simulink model "lookup_nD_TestGen33"  (R2017b)
settings: Solver=FixedStepDiscrete  StartTime=0.0  StopTime=10.0  RelTol=1e-3
model workspace (MAT data in the model file):
  LUTObjLKnD33 = Simulink.LookupTable
  LUTObjLKnD33.Table = Simulink.lookuptable.Table
  LUTObjLKnD33.Table.Value = reshape([4 16 10 4 16 10 4 16 10 4 16 10 4 16 10 4 16 10 5 19 18 5 19 18 5 19 18 5 19 18 5 19 18 5 19 18 6 20 23 6 20 23 6 20 23 6 20 23 6 20 23 6 20 23 7 21 24 7 21 24 7 21 24 7 21 24 7 21 24 7 21 24 8 22 25 8 22 25 8 22 25 8 22 25 8 22 25 8 22 25 4 16 10 4 16 10 4 16 10 4 16 10 4 16 10 4 16 10 5 19 18 5 19 18 5 19 18 5 19 18 5 19 18 5 19 18 6 20 23 6 20 23 6 20 23 6 20 23 6 20 23 6 20 23 7 21 24 7 21 24 7 21 24 7 21 24 7 21 24 7 21 24 8 22 25 8 22 25 8 22 25 8 22 25 8 22 25 8 22 25 4 16 10 4 16 10 4 16 10 4 16 10 4 16 10 4 16 10 5 19 18 5 19 18 5 19 18 5 19 18 5 19 18 5 19 18 6 20 23 6 20 23 6 20 23 6 20 23 6 20 23 6 20 23 7 21 24 7 21 24 7 21 24 7 21 24 7 21 24 7 21 24 8 22 25 8 22 25 8 22 25 8 22 25 8 22 25 8 22 25 4 16 10 4 16 10 4 16 10 4 16 10 4 16 10 4 16 10 5 19 18 5 19 18 5 19 18 5 19 18 5 19 18 5 19 18 6 20 23 6 20 23 6 20 23 6 20 23 6 20 23 6 20 23 7 21 24 7 21 24 7 21 24 7 21 24 7 21 24 7 21 24 8 22 25 8 22 25 8 22 25 8 22 25 8 22 25 8 22 25 4 16 10 4 16 10 4 16 10 4 16 10 4 16 10 4 16 10 5 19 18 5 19 18 5 19 18 5 19 18 5 19 18 5 19 18 6 20 23 6 20 23 6 20 23 6 20 23 6 20 23 6 20 23 7 21 24 7 21 24 7 21 24 7 21 24 7 21 24 7 21 24 8 22 25 8 22 25 8 22 25 8 22 25 8 22 25 8 22 25 4 16 10 4 16 10 4 16 10 4 16 10 4 16 10 4 16 10 5 19 18 5 19 18 5 19 18 5 19 18 5 19 18 5 19 18 6 20 23 6 20 23 6 20 23 6 20 23 6 20 23 6 20 23 7 21 24 7 21 24 7 21 24 7 21 24 7 21 24 7 21 24 8 22 25 8 22 25 8 22 25 8 22 25 8 22 25 8 22 25 4 16 10 4 16 10 4 16 10 4 16 10 4 16 10 4 16 10 5 19 18 5 19 18 5 19 18 5 19 18 5 19 18 5 19 18 6 20 23 6 20 23 6 20 23 6 20 23 6 20 23 6 20 23 7 21 24 7 21 24 7 21 24 7 21 24 7 21 24 7 21 24 8 22 25 8 22 25 8 22 25 8 22 25 8 22 25 8 22 25 4 16 10 4 16 10 4 16 10 4 16 10 4 16 10 4 16 10 5 19 18 5 19 18 5 19 18 5 19 18 5 19 18 5 19 18 6 20 23 6 20 23 6 20 23 6 20 23 6 20 23 6 20 23 7 21 24 7 21 24 7 21 24 7 21 24 7 21 24 7 21 24 8 22 25 8 22 25 8 22 25 8 22 25 8 22 25 8 22 25], [2 5 3 2 3 4])
  LUTObjLKnD33.Table.Dimensions = [2 5 3 2 3 4]
  LUTObjLKnD33.Table.DataType = 'double'
  LUTObjLKnD33.Table.FieldName = 'Table'
  LUTObjLKnD33.Breakpoints(1) = Simulink.lookuptable.Breakpoint
  LUTObjLKnD33.Breakpoints(1).Value = [55.1141389852; 115.959753023]
  LUTObjLKnD33.Breakpoints(1).TunableSizeName = 'N1'
  LUTObjLKnD33.Breakpoints(1).Dimensions = [2 1]
  LUTObjLKnD33.Breakpoints(1).DataType = 'double'
  LUTObjLKnD33.Breakpoints(1).FieldName = 'BP1'
  LUTObjLKnD33.Breakpoints(2) = Simulink.lookuptable.Breakpoint
  LUTObjLKnD33.Breakpoints(2).Value = [7.76812849772; 29.4671423139; 31.4118384647; 67.8975675265; 99.4838661864]
  LUTObjLKnD33.Breakpoints(2).TunableSizeName = 'N2'
  LUTObjLKnD33.Breakpoints(2).Dimensions = [5 1]
  LUTObjLKnD33.Breakpoints(2).DataType = 'double'
  LUTObjLKnD33.Breakpoints(2).FieldName = 'BP2'
  LUTObjLKnD33.Breakpoints(3) = Simulink.lookuptable.Breakpoint
  LUTObjLKnD33.Breakpoints(3).Value = [61.8687772676; 86.0025709843; 101.597469424]
  LUTObjLKnD33.Breakpoints(3).TunableSizeName = 'N3'
  LUTObjLKnD33.Breakpoints(3).Dimensions = [3 1]
  LUTObjLKnD33.Breakpoints(3).DataType = 'double'
  LUTObjLKnD33.Breakpoints(3).FieldName = 'BP3'
  LUTObjLKnD33.Breakpoints(4) = Simulink.lookuptable.Breakpoint
  LUTObjLKnD33.Breakpoints(4).Value = [45.1909970892; 88.5981999607]
  LUTObjLKnD33.Breakpoints(4).TunableSizeName = 'N4'
  LUTObjLKnD33.Breakpoints(4).Dimensions = [2 1]
  LUTObjLKnD33.Breakpoints(4).DataType = 'double'
  LUTObjLKnD33.Breakpoints(4).FieldName = 'BP4'
  LUTObjLKnD33.Breakpoints(5) = Simulink.lookuptable.Breakpoint
  LUTObjLKnD33.Breakpoints(5).Value = [48.7941996351; 67.4387180631; 70.5577350792]
  LUTObjLKnD33.Breakpoints(5).TunableSizeName = 'N5'
  LUTObjLKnD33.Breakpoints(5).Dimensions = [3 1]
  LUTObjLKnD33.Breakpoints(5).DataType = 'double'
  LUTObjLKnD33.Breakpoints(5).FieldName = 'BP5'
  LUTObjLKnD33.Breakpoints(6) = Simulink.lookuptable.Breakpoint
  LUTObjLKnD33.Breakpoints(6).Value = [9.10881332364; 75.0691190596; 86.3387833349; 95.4088639299]
  LUTObjLKnD33.Breakpoints(6).TunableSizeName = 'N6'
  LUTObjLKnD33.Breakpoints(6).Dimensions = [4 1]
  LUTObjLKnD33.Breakpoints(6).DataType = 'double'
  LUTObjLKnD33.Breakpoints(6).FieldName = 'BP6'
  LUTObjLKnD33.SupportTunableSize = 0
  LUTObjLKnD33.StructTypeInfo = Simulink.lookuptable.StructTypeInfo
  LUTObjLKnD33.StructTypeInfo.Name = 'LUT'
  LUTObjLKnD33.StructTypeInfo.DataScope = 'Auto'
settings Model: Creator=ktrinh  LastModifiedBy=ktrinh
settings DebuggingCC: ParameterOverflowMsg=none

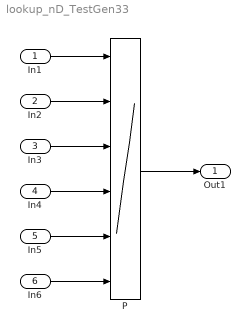
== system lookup_nD_TestGen33 ==
  In1 : Inport  OutMin=0  OutMax=127  PortDimensions=3
  In2 : Inport  Port=2  OutMin=0  OutMax=127
  In3 : Inport  Port=3  OutMin=0  OutMax=127
  In4 : Inport  Port=4  OutMin=0  OutMax=127
  In5 : Inport  Port=5  OutMin=0  OutMax=127
  In6 : Inport  Port=6  OutMin=0  OutMax=127
  P : Lookup_n-D  NumberOfTableDimensions=6  DataSpecification=Lookup table object  LookupTableObject=LUTObjLKnD33  BreakpointsForDimension3=[5, 7]  Table=reshape(repmat([4 5 6;16 19 20;10 18 23],1,2),[3,3,2])  InterpMethod=Nearest  ExtrapMethod=Clip  InternalRulePriority=Speed  OutDataTypeStr=double  RndMeth=Simplest  SaturateOnIntegerOverflow=on  InputSameDT=on
  Out1 : Outport
  wires:
  In1/1 -> P/1
  In2/1 -> P/2
  In3/1 -> P/3
  In4/1 -> P/4
  In5/1 -> P/5
  In6/1 -> P/6
  P/1 -> Out1/1
